simulink model "problem_1_sim"  (R2025a)
settings: Solver=VariableStepAuto  StartTime=0.0  StopTime=t_sim  RelTol=1e-3
values from neighbouring files (symbols this model uses):
  C = [1 0]    [problem_2.m]
  K = dlqr(Aaug,Baug,Q,R)    [problem_2.m]
  Ts = 0.05    [problem_2.m]
libraries: cstblocks x1
settings Model: Creator=s360159  LastModifiedBy=s360159

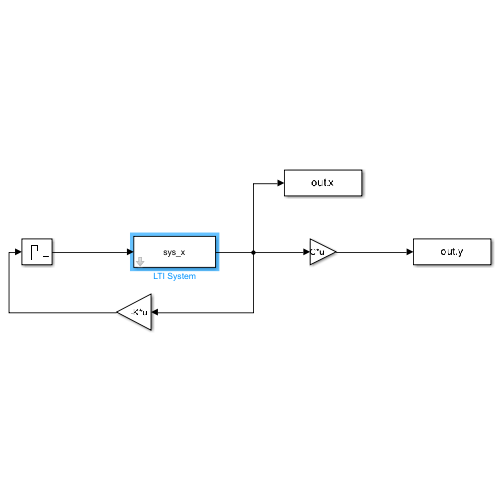
[thumbnail: Simulink's stored preview of the top-level diagram]
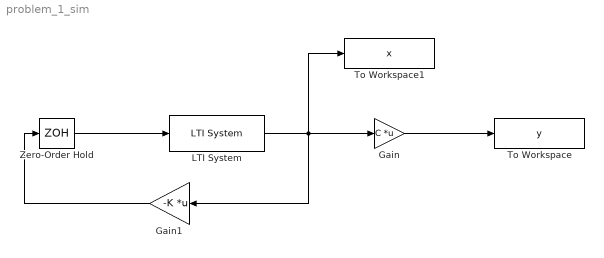
== system problem_1_sim ==
  Gain : Gain  Gain=C  Multiplication=Matrix(K*u)
  Gain1 : Gain  Gain=-K  Multiplication=Matrix(K*u)
  LTI System : cstblocks/LTI System  sys=sys_x  IC=x0  PadeOrder=0
  To Workspace : ToWorkspace  VariableName=y  SaveFormat=Timeseries  SampleTime=Ts
  To Workspace1 : ToWorkspace  VariableName=x  SaveFormat=Timeseries  SampleTime=Ts
  Zero-Order Hold : ZeroOrderHold  SampleTime=-1
  wires:
  Zero-Order Hold/1 -> LTI System/1
  LTI System/1 -> To Workspace1/1, Gain1/1, Gain/1
  Gain/1 -> To Workspace/1
  Gain1/1 -> Zero-Order Hold/1
